simulink model "Robot (1)"  (R2019a)
settings: Solver=ode3  StartTime=0.0  StopTime=100.0  FixedStep=0.01  RelTol=1e-3
undefined symbols (not defined in the file or in its folder): DiscIntNeverNeededParam
libraries: simulink x1
settings Model: EnablePacing=on  Creator=Alex  LastModifiedBy=Alex
settings DataIOCC: ReturnWorkspaceOutputs=off

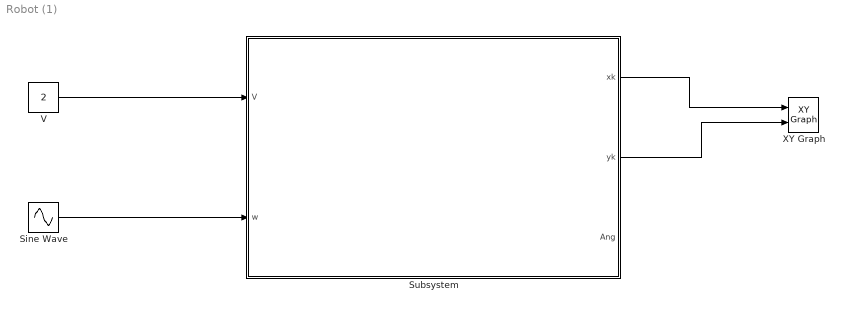
== system Robot (1) ==
  Sine Wave : Sin  Amplitude=10  Frequency=10  SampleTime=0
  Subsystem : Subsystem
  V : Constant  Value=2
  XY Graph : simulink/Sinks/XY Graph  xmin=-5  xmax=10  ymin=-10  ymax=10  st=0.01
  wires:
  V/1 -> Subsystem/1(V)
  Sine Wave/1 -> Subsystem/2("w ")
  Subsystem/1(xk) -> XY Graph/1
  Subsystem/2(yk) -> XY Graph/2

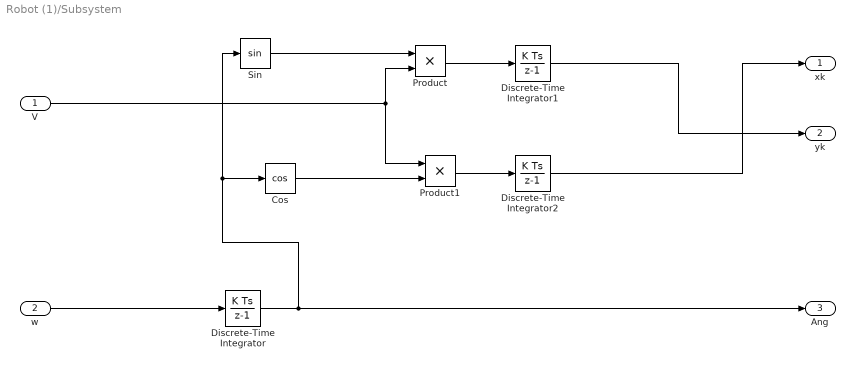
== system Robot (1)/Subsystem ==
  V : Inport
  "w " : Inport  Port=2
  Cos : Trigonometry  Operator=cos
  Discrete-Time Integrator : DiscreteIntegrator  SampleTime=0.01  ICPrevOutput=DiscIntNeverNeededParam  ICPrevScaledInput=DiscIntNeverNeededParam
  Discrete-Time Integrator1 : DiscreteIntegrator  InitialCondition=-4  SampleTime=-1  ICPrevOutput=DiscIntNeverNeededParam  ICPrevScaledInput=DiscIntNeverNeededParam
  Discrete-Time Integrator2 : DiscreteIntegrator  InitialCondition=-4  SampleTime=-1  ICPrevOutput=DiscIntNeverNeededParam  ICPrevScaledInput=DiscIntNeverNeededParam
  Product : Product
  Product1 : Product
  Sin : Trigonometry
  xk : Outport
  yk : Outport  Port=2
  Ang : Outport  Port=3
  wires:
  Sin/1 -> Product/1
  Cos/1 -> Product1/2
  V/1 -> Product1/1, Product/2
  Product/1 -> Discrete-Time Integrator1/1
  Discrete-Time Integrator2/1 -> xk/1
  Discrete-Time Integrator1/1 -> yk/1
  Product1/1 -> Discrete-Time Integrator2/1
  "w "/1 -> Discrete-Time Integrator/1
  Discrete-Time Integrator/1 -> Ang/1, Cos/1, Sin/1
